simulink model "clock_recovery_4"  (Simulink 7.4)
settings: Solver=ode45  StartTime=0.0  StopTime=1e-5  MaxStep=.1/bit_rate  RelTol=1e-3
PreLoadFcn:
  | bit_rate=2e9;   % bits per second
  | load diff_backplane_model;
undefined symbols (not defined in the file or in its folder): RationalFuncModel
libraries: simulink x8, dspsigattribs x8, dspsigops x6, commblksprivate x4, dspstat3 x2, commrandsrc2 x1, dspbuff3 x1, dspsnks4 x1
settings Model: Creator=dbenson  LastModifiedBy=Dick
settings SolverCC: ZeroCrossControl=EnableAll
settings OptimizationCC: InitFltsAndDblsToZero=on

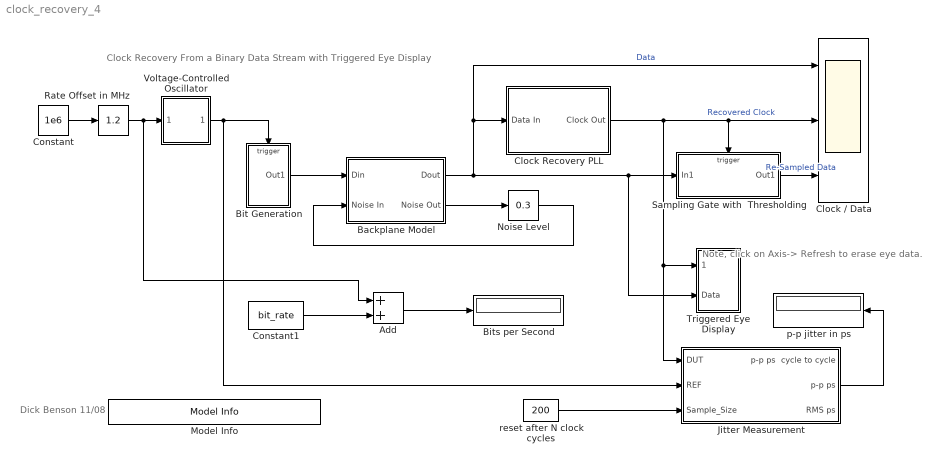
== system clock_recovery_4 ==
  note: Clock Recovery From a Binary Data Stream
      | with
      | Triggered Eye Display
  note: Note, click on Axis-> Refresh
      | to erase eye data.
  note: Dick Benson
      | 11/08
  Add : Sum  OutDataType=sfix(16)  OutScaling=2^-10
  Backplane Model : Subsystem
  Bit Generation : Subsystem
  Bits per Second : Display
  "Clock / Data " : Scope  NumInputPorts=3
      settings: TimeRange=1e-009  YMin=-1~-0.2~-0.2  YMax=1~1.2~1.2
  Clock Recovery PLL : Subsystem
  Constant : Constant  Value=1e6  OutDataType=sfix(16)  OutScaling=2^0
  Constant1 : Constant  Value=bit_rate  OutDataType=sfix(16)  OutScaling=2^0
  "Jitter Measurement " : Subsystem
  Model Info : simulink/Model-Wide Utilities/Model Info  SystemSampleTime=-1  InitialBlockCM=None  BlockCM=None  Frame=on  DisplayStringWithTags=Copywrite 2008-2010 The MathWorks, Inc.  HorizontalTextAlignment=Center  LeftAlignmentValue=0.5  SourceBlockDiagram=clock_recovery_4  TagMaxNumber=20
  Noise Level : simulink/Math Operations/Slider Gain  SystemSampleTime=-1  low=0  gain=0.3  high=1
  Rate Offset in MHz : simulink/Math Operations/Slider Gain  SystemSampleTime=-1  low=-5  gain=1.2  high=5
  Sampling Gate with  Thresholding : Subsystem
  Triggered Eye Display : Subsystem
  Voltage-Controlled Oscillator : Subsystem  mask(Voltage-Controlled Oscillator){Ac=1, Fc=bit_rate, Kc=1, Ph=0}
      mask prompts: Ac "Output amplitude:"; Fc "Oscillation frequency (Hz):"; Kc "Input sensitivity:"; Ph "Initial phase (rad):"
      mask help: Generate a continuous-time output signal whose frequency changes in response to the amplitude variations of the input signal. The input signal must be a sample-based scalar.
      mask init:
      | if ((length(Ac)~=1) | (length(Fc)~=1) | (length(Ph)~=1) | (length(Kc)~=1) )error('Mask parameters must be scalar values.');end;
      | pi2=2*pi;
      mask Help: helpview(commbhelp)
      mask Display: disp('VCO')
  p-p jitter in ps : Display
  reset after N clock cycles : Constant  Value=200  VectorParams1D=off  OutDataType=sfix(16)  OutScaling=2^0
  wires:
  Clock Recovery PLL/1(Clock Out) -> Sampling Gate with  Thresholding/Trigger, "Clock / Data "/2, Triggered Eye Display/1(Trigger), "Jitter Measurement "/1(DUT)  "Recovered Clock"
  Bit Generation/1(Out1) -> Backplane Model/1(Din)
  Backplane Model/1(Dout) -> Clock Recovery PLL/1(Data In), "Clock / Data "/1, Sampling Gate with  Thresholding/1(In1), Triggered Eye Display/2(Data)  "Data"
  Sampling Gate with  Thresholding/1(Out1) -> "Clock / Data "/3  "Re-Sampled Data"
  Add/1 -> Bits per Second/1
  "Jitter Measurement "/2(p-p ps) -> p-p jitter in ps/1
  reset after N clock cycles/1 -> "Jitter Measurement "/3(Sample_Size)
  Backplane Model/2(Noise Out) -> Noise Level/1
  Noise Level/1 -> Backplane Model/2(Noise In)
  Voltage-Controlled Oscillator/1(out_1) -> Bit Generation/Trigger, "Jitter Measurement "/2(REF)
  Rate Offset in MHz/1 -> Voltage-Controlled Oscillator/1(in_1), Add/1
  Constant/1 -> Rate Offset in MHz/1
  Constant1/1 -> Add/2

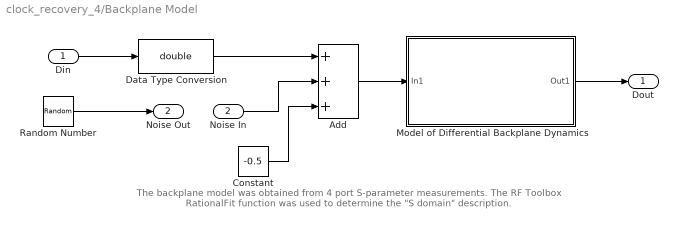
== system clock_recovery_4/Backplane Model ==
  note: The backplane model was obtained from 4 port S-parameter measurements.
      | The RF Toolbox RationalFit function was used to determine the "S domain"
      | description.
  Din : Inport
  Noise In : Inport  Port=2
  Add : Sum  Inputs=+++  OutDataType=sfix(16)  OutScaling=2^-10
  Constant : Constant  Value=-0.5  OutDataType=sfix(16)  OutScaling=2^0
  Data Type Conversion : DataTypeConversion  OutDataTypeMode=double  OutDataType=sfix(16)  OutScaling=2^0  OutDataTypeStr=double
  Model of Differential Backplane Dynamics : Subsystem  mask{RationalFuncModel=RationalFuncModel}
      mask prompts: RationalFuncModel "Rational Model"
      mask init:
      | nPoles = length(RationalFuncModel.A);
      | OriginalA = RationalFuncModel.A; OriginalC = RationalFuncModel.C;
      | A = zeros(length(OriginalA), 1); C = zeros(length(OriginalC), 1);
      | kk = 1;
      | for k = 1:nPoles
      |     if isnan(OriginalA(k))
      |         continue
      |     elseif ~isreal(OriginalA(k))
      |         % Complex poles and residues
      |         pos = find(OriginalA == conj(OriginalA(k)), 1);
      |         OriginalA(pos) = NaN; OriginalC(pos) = NaN;
      |     end
      |     A(kk) = OriginalA(k); C(kk) = OriginalC(k); kk = kk + 1;
      | end
      | A = A(1:kk-1); C = C(1:kk-1);
      | % Get the Numerators and Denominators of the Laplace Transform S-Domain Filters
      | % Convert the vectors of real and complex poles and residues of the rational function model 
      | % into real numerators and denominators of Laplace Transform S-domain filters. 
      | 
      | nA = length(A); 
      | rat_den = cell(nA, 1); 
      | rat_num = cell(nA, 1);
      | 
      | 
      | for k = 1:nA
      |     if isreal(A(k))     % Real poles
      |         rat_num{k} = C(k); rat_den{k} = [1, -A(k)];
      |     else                % Complex poles
      |         real_a = real(A(k)); imag_a = imag(A(k));
      |         real_c = real(C(k)); imag_c = imag(C(k));
      |         rat_num{k} = [2*real_c, -2*(real_a*real_c+imag_a*imag_c)];
      |         rat_den{k} = [1, -2*real_a, real_a^2+imag_a^2];
      |     end
      | end
      | xfer_blocks = length(rat_den);
      | rtsys        = gcb;   % Block become "current" when its initialize function is called.
      | Xfer_stages  = find_system(rtsys,'RegExp','on','lookUnderMasks', 'all', 'FollowLinks','on','BlockType','TransferFcn'); % note there are no spaces in the TransferFcn !!!
      | L_stage = length(Xfer_stages);
      |    %In_port      = find_system(rtsys,'lookUnderMasks', 'all','BlockType','Inport');
      |    %Out_port     = find_system(rtsys,'lookUnderMasks', 'all','BlockType','Outport');
      |    Gain_stage   = find_system(rtsys,'lookUnderMasks', 'all', 'BlockType','Gain');
      |    Sum_stages   = find_system(rtsys,'lookUnderMasks', 'all', 'BlockType','Sum');
      |    Delay_stage  = find_system(rtsys,'lookUnderMasks', 'all', 'BlockType','TransportDelay');
      | 
      | if L_stage ~=nA
      |   %  Delete existing elements (Brute Force!) 
      |    disp('Programatically Building Rational Transfer Function Block ') 
      |   % need to rebuild the model
      |    if L_stage >1
      |        for k=2:L_stage
      |            % need to go in order that is in Xfer_stages
      |            s = Xfer_stages{k};
      |            p = findstr('_',s);
      |            p_last = p(end);
      |            stage=(s((p_last+1):end));
      |            delete_line(rtsys, 'In1/1' , ['stage_',stage,'/1']);
      |            delete_line(rtsys,['stage_',stage,'/1'],['Combiner/',stage]);
      |            % disp(['Deleting ',['stage_',stage]])
      |            delete_block(Xfer_stages{k}); 
      |            drawnow;
      |        end;
      |    end;
      | 
      |    
      |    % set direct feedthrough gain
      |    set_param(Gain_stage{1},'Gain',sprintf('%30d',RationalFuncModel.D)); % the gain value
      |    % set delay element value
      |    % get_param(Delay_stage{1},'ObjectParameters')
      |    set_param(Delay_stage{1},'Delay',sprintf('%30d',RationalFuncModel.Delay)); % delay value
      |    set_param(Delay_stage{1},'BufferSize','2*6144'); % this needs more work ##############
      |    drawnow;
      |    
      |    
      |    % Rebuild structure
      |    % setup combiner (summer) to correct number of inputs
      |    % Set up the Combiner
      |    % get_param(Sum_stages{2},'ObjectParameters')
      |    % get_param(Sum_stages{2},'Inputs')
      |    s='+';
      |    for k=2:xfer_blocks
      |        s=[s,'+'];
      |    end;
      |    set_param(Sum_stages{2},'Inputs',s);  % sets number of inputs to Combiner block
      | 
      |    % add Xfer Fcn blocks
      |    % get_param(Xfer_stages{1},'ObjectParameters')
      |    xfer_pos=get_param(Xfer_stages{1},'Position');
      |    % name_1 = get_param(Xfer_stages{1},'Name');
      |    nstring = ['[',sprintf('%35.5f',rat_num{1}),']'];
      |    dstring = ['[',sprintf('%35.5f',rat_den{1}),']'];
      |    set_param(Xfer_stages{1},'Numerator',nstring,'Denominator',dstring);
      |    src = Xfer_stages{1};  % use as reference block
      |    for k=2:xfer_blocks
      |        dst=[src(1:(end-1)),int2str(k)];
      |        nstring = ['[',sprintf('%35.5f',rat_num{k}),']'];
      |        dstring = ['[',sprintf('%35.5f',rat_den{k}),']'];
      |        add_block(src,dst,'Position',[xfer_pos(1) ,xfer_pos(2)+(k-1)*50, xfer_pos(3) ,xfer_pos(4)+(k-1)*50],'Numerator',nstring,'Denominator',dstring);
      |        add_line(rtsys,'In1/1',['stage_',int2str(k),'/1'],'autorouting','on'); % hook up inputs
      |        add_line(rtsys,['stage_',int2str(k),'/1'],['Combiner/',int2str(k)],'autorouting','on'); % and outputs 
      |     end;
      | 
      | else
      |     % Order has not changed, but coefficients may have.
      |     disp('No programatic build is required, but coefficients are being updated.')
      |     % set direct feedthrough gain
      |     set_param(Gain_stage{1},'Gain',sprintf('%30d',RationalFuncModel.D)); % the gain value
      |     % set delay element value
      |     set_param(Delay_stage{1},'Delay',sprintf('%30d',RationalFuncModel.Delay)); % delay value
      |     set_param(Delay_stage{1},'BufferSize','2*6144'); % this needs more work ##############
      |     
      |     src = Xfer_stages{1};  % use as reference block
      |     for k=1:xfer_blocks
      |        dst=[src(1:(end-1)),int2str(k)];
      |        nstring = ['[',sprintf('%35.5f',rat_num{k}),']'];
      |        dstring = ['[',sprintf('%35.5f',rat_den{k}),']'];
      |        set_param(dst,'Numerator',nstring,'Denominator',dstring); drawnow;
      |     end;
      |         
      | end;
      mask Display: disp('S domain \n Rational Transfer Function Model \n Do Not Edit This Subsystem!')
  Random Number : RandomNumber  SampleTime=0
  Dout : Outport
  Noise Out : Outport  Port=2
  wires:
  Din/1 -> Data Type Conversion/1
  Add/1 -> Model of Differential Backplane Dynamics/1(In1)
  Data Type Conversion/1 -> Add/1
  Model of Differential Backplane Dynamics/1(Out1) -> Dout/1
  Random Number/1 -> Noise Out/1
  Noise In/1 -> Add/2
  Constant/1 -> Add/3

== system clock_recovery_4/Bit Generation ==
  Trigger : TriggerPort
  Bernoulli Binary Generator : commrandsrc2/Bernoulli Binary Generator  DialogController=commDDGCreate  DialogControllerArgs=DataTag0  SystemSampleTime=-1  P=0.5  seed=21  Ts=-1  frameBased=off  sampPerFrame=1  orient=off  outDataType=boolean
  Out1 : Outport
  wires:
  Bernoulli Binary Generator/1 -> Out1/1

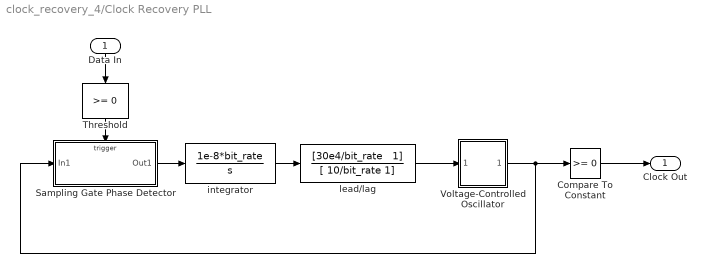
== system clock_recovery_4/Clock Recovery PLL ==
  Data In : Inport
  Compare To Constant : simulink/Logic and Bit Operations/Compare To Constant  SystemSampleTime=-1  relop=>=  const=0  LogicOutDataTypeMode=boolean  ZeroCross=off
  Sampling Gate Phase Detector : Subsystem
  Threshold : simulink/Logic and Bit Operations/Compare To Constant  SystemSampleTime=-1  relop=>=  const=0  LogicOutDataTypeMode=boolean  ZeroCross=off
  Voltage-Controlled Oscillator : Subsystem  mask(Voltage-Controlled Oscillator){Ac=1, Fc=bit_rate, Kc=bit_rate, Ph=0}
      mask prompts: Ac "Output amplitude:"; Fc "Oscillation frequency (Hz):"; Kc "Input sensitivity:"; Ph "Initial phase (rad):"
      mask help: Generate a continuous-time output signal whose frequency changes in response to the amplitude variations of the input signal. The input signal must be a sample-based scalar.
      mask init:
      | if ((length(Ac)~=1) | (length(Fc)~=1) | (length(Ph)~=1) | (length(Kc)~=1) )error('Mask parameters must be scalar values.');end;
      | pi2=2*pi;
      mask Help: helpview(commbhelp)
      mask Display: disp('VCO')
  integrator : TransferFcn  Numerator=1e-8*bit_rate  Denominator=[1 0]
  lead/lag : TransferFcn  Numerator="[30e4/bit_rate   1]"  Denominator=[ 10/bit_rate 1]
  Clock Out : Outport
  wires:
  lead/lag/1 -> Voltage-Controlled Oscillator/1(in_1)
  Voltage-Controlled Oscillator/1(out_1) -> Sampling Gate Phase Detector/1(In1), Compare To Constant/1
  integrator/1 -> lead/lag/1
  Sampling Gate Phase Detector/1(Out1) -> integrator/1
  Threshold/1 -> Sampling Gate Phase Detector/Trigger
  Data In/1 -> Threshold/1
  Compare To Constant/1 -> Clock Out/1

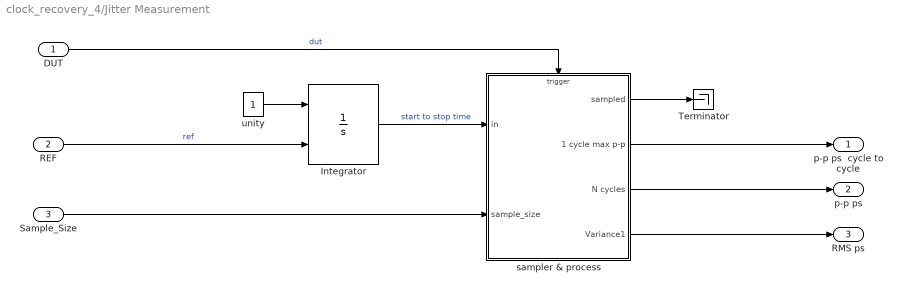
== system clock_recovery_4/Jitter Measurement  ==
  DUT : Inport  OutDataType=sfix(16)  OutScaling=2^0
  REF : Inport  Port=2  OutDataType=sfix(16)  OutScaling=2^0
  Sample_Size : Inport  Port=3  OutDataType=sfix(16)  OutScaling=2^0
  Integrator : Integrator  ExternalReset=rising
  Terminator : Terminator
  sampler & process : Subsystem  TreatAsAtomicUnit=on
  unity : Constant  OutDataTypeMode=double  OutDataType=sfix(16)  OutScaling=2^0  OutDataTypeStr=double
  p-p ps  cycle to cycle : Outport  OutDataType=sfix(16)  OutScaling=2^0
  p-p ps : Outport  Port=2  OutDataType=sfix(16)  OutScaling=2^0
  RMS ps : Outport  Port=3  OutDataType=sfix(16)  OutScaling=2^0
  wires:
  DUT/1 -> sampler & process/Trigger  "dut"
  REF/1 -> Integrator/2  "ref"
  Integrator/1 -> sampler & process/1(in)  "start to stop time"
  Sample_Size/1 -> sampler & process/2(sample_size)
  sampler & process/3(N cycles) -> p-p ps/1
  sampler & process/4(Variance1) -> RMS ps/1
  unity/1 -> Integrator/1
  sampler & process/2(1 cycle max p-p) -> p-p ps  cycle to cycle/1
  sampler & process/1(sampled) -> Terminator/1

== system clock_recovery_4/Sampling Gate with  Thresholding ==
  In1 : Inport  OutDataType=sfix(16)  OutScaling=2^0
  Trigger : TriggerPort
  Compare To Constant : simulink/Logic and Bit Operations/Compare To Constant  SystemSampleTime=-1  relop=>=  const=0  LogicOutDataTypeMode=boolean  ZeroCross=off
  Out1 : Outport  OutDataType=sfix(16)  OutScaling=2^0
  wires:
  In1/1 -> Compare To Constant/1
  Compare To Constant/1 -> Out1/1

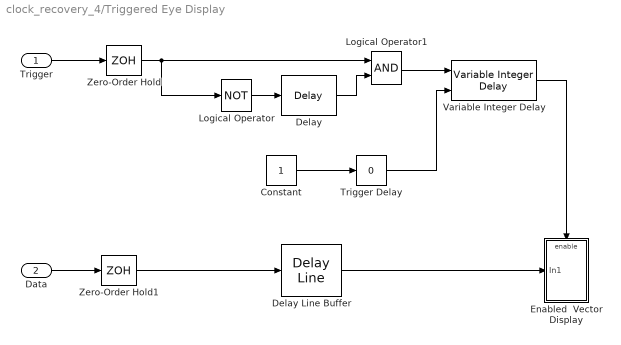
== system clock_recovery_4/Triggered Eye Display ==
  Trigger : Inport
  Data : Inport  Port=2
  Constant : Constant  OutDataType=sfix(16)  OutScaling=2^0
  Delay : dspsigops/Delay  dly_unit=Samples  delay=1  ic_detail=off  dif_ic_for_ch=off  dif_ic_for_dly=off  ic=0  reset_popup=None
  Delay Line Buffer : dspbuff3/Delay Line  siz=200  ic=0  directfeed=off  enable_output=off  hold_output=off
  Enabled  Vector Display : Subsystem
  Logical Operator : Logic  Operator=NOT  AllPortsSameDT=off  OutDataTypeMode=boolean  OutDataTypeStr=boolean
  Logical Operator1 : Logic  AllPortsSameDT=off  OutDataTypeMode=boolean  OutDataTypeStr=boolean
  Trigger Delay : simulink/Math Operations/Slider Gain  SystemSampleTime=-1  low=0  gain=0  high=100
  Variable Integer Delay : dspsigops/Variable Integer Delay  dmax=100  ic=0  noDFT=off
  Zero-Order Hold : ZeroOrderHold  SampleTime=.01/bit_rate
  Zero-Order Hold1 : ZeroOrderHold  SampleTime=.01/bit_rate
  wires:
  Zero-Order Hold/1 -> Logical Operator1/1, Logical Operator/1
  Logical Operator/1 -> Delay/1
  Delay/1 -> Logical Operator1/2
  Trigger/1 -> Zero-Order Hold/1
  Data/1 -> Zero-Order Hold1/1
  Zero-Order Hold1/1 -> Delay Line Buffer/1
  Delay Line Buffer/1 -> Enabled  Vector Display/1(In1)
  Logical Operator1/1 -> Variable Integer Delay/1
  Variable Integer Delay/1 -> Enabled  Vector Display/Enable
  Trigger Delay/1 -> Variable Integer Delay/2
  Constant/1 -> Trigger Delay/1

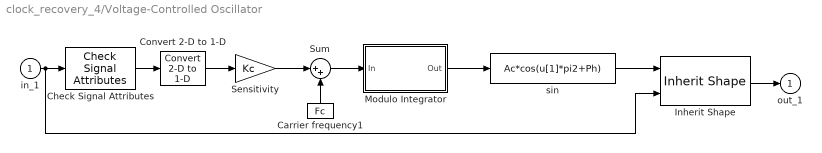
== system clock_recovery_4/Voltage-Controlled Oscillator ==
  in_1 : Inport  OutDataType=sfix(16)  OutScaling=2^0
  Carrier frequency1 : Constant  Value=Fc  OutDataType=sfix(16)  OutScaling=2^0
  Check Signal Attributes : dspsigattribs/Check Signal Attributes  SystemSampleTime=-1  SigAttribCheckMethod=Does not match attributes exactly  Complexity=Ignore  Frame=Sample-based  DimsCheckMethod=Is...  Dimensions=Scalar (1-D or 2-D)  DatatypeCheckMethod=Ignore  DatatypeGeneral=Boolean  DtypeFloatSpecific=Any floating-point  DtypeFixedSpecific=Any fixed-point  DtypeIntSpecific=Any integer  SampleMode=Ignore
  Convert 2-D to 1-D : dspsigattribs/Convert 2-D to 1-D  SystemSampleTime=-1
  Inherit Shape : commblksprivate/Inherit Shape
  Modulo Integrator : Subsystem  mask(Modulo Integrator){modu=1, init=0}
      mask prompts: modu "Absolute value bound:"; init "Initial condition:"
      mask help:
      | Integrate the input signal in continuous time and then uses the Absolute value bound parameter, K, to produce output strictly between -K and K. The block uses the rem function in MATLAB.
      |
      | The input must be sample-based.
      mask init:
      | [modu, init]=commblkmodint(gcb);
      mask Help: helpview(commbhelp)
      mask Display: disp('Modulo\nIntegrator')
  Sensitivity : Gain  Gain=Kc  ParameterDataType=sfix(16)  ParameterScaling=2^0  OutDataType=sfix(16)  OutScaling=2^0  SaturateOnIntegerOverflow=on  OutDataTypeStr=Inherit: Same as input  ParamDataTypeStr=Inherit: Same as input
  Sum : Sum  Inputs=|++  OutDataType=sfix(16)  OutScaling=2^0  SaturateOnIntegerOverflow=on  InputSameDT=on  OutDataTypeStr=Inherit: Same as first input
  sin : Fcn  Expr=Ac*cos(u[1]*pi2+Ph)
  out_1 : Outport  OutDataType=sfix(16)  OutScaling=2^0  InitialOutput=0
  wires:
  Check Signal Attributes/1 -> Convert 2-D to 1-D/1
  Inherit Shape/1 -> out_1/1
  sin/1 -> Inherit Shape/1
  Convert 2-D to 1-D/1 -> Sensitivity/1
  in_1/1 -> Check Signal Attributes/1, Inherit Shape/2
  Sensitivity/1 -> Sum/1
  Carrier frequency1/1 -> Sum/2
  Modulo Integrator/1(Out) -> sin/1
  Sum/1 -> Modulo Integrator/1(In)

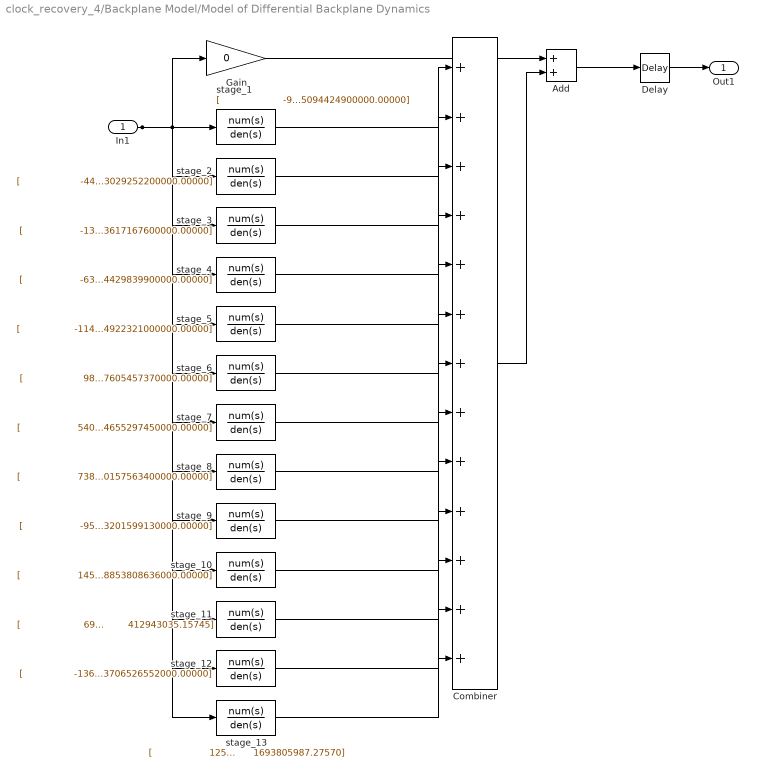
== system clock_recovery_4/Backplane Model/Model of Differential Backplane Dynamics ==
  In1 : Inport  OutDataType=sfix(16)  OutScaling=2^0
  Add : Sum  OutDataType=sfix(16)  OutScaling=2^-10
  Combiner : Sum  Inputs=+++++++++++++  OutDataType=sfix(16)  OutScaling=2^-10
  Delay : TransportDelay  DelayTime=5.950332e-009  BufferSize=2*6144
  Gain : Gain  Gain=0  ParameterDataType=sfix(16)  ParameterScaling=2^0  OutDataType=sfix(16)  OutScaling=2^0
  stage_1 : TransferFcn  Numerator="[                     -9788555.30433           327601364005149500.00000]"  Denominator="[                            1.00000                   1329591272.34003       5044242645094424900000.00000]"
  stage_10 : TransferFcn  Numerator="[                   1459155273.40124         16659733674469984000.00000]"  Denominator="[                            1.00000                   4539756715.10415         55819688853808636000.00000]"
  stage_11 : TransferFcn  Numerator="[                     69890645.34105]"  Denominator="[                            1.00000                    412943035.15745]"
  stage_12 : TransferFcn  Numerator="[                 -13652042138.80265        -20558972237464187000.00000]"  Denominator="[                            1.00000                   6618433668.53674         16544543706526552000.00000]"
  stage_13 : TransferFcn  Numerator="[                   1252271665.41653]"  Denominator="[                            1.00000                   1693805987.27570]"
  stage_2 : TransferFcn  Numerator="[                    -44020735.77568          2540524038618086400.00000]"  Denominator="[                            1.00000                   3458566159.00361       3748760873029252200000.00000]"
  stage_3 : TransferFcn  Numerator="[                   -134087089.17792          1299068138817301200.00000]"  Denominator="[                            1.00000                   4003736859.07552       2889729443617167600000.00000]"
  stage_4 : TransferFcn  Numerator="[                   -637966669.86598         -4277202848730946600.00000]"  Denominator="[                            1.00000                   7795187757.93497       1980584994429839900000.00000]"
  stage_5 : TransferFcn  Numerator="[                  -1141903615.08100        -42517650479109677000.00000]"  Denominator="[                            1.00000                   6993651024.28011       1349862304922321000000.00000]"
  stage_6 : TransferFcn  Numerator="[                    985358456.83414        -87067793597322330000.00000]"  Denominator="[                            1.00000                   7852217292.40317        928900427605457370000.00000]"
  stage_7 : TransferFcn  Numerator="[                   5400452167.19306        -32568397331195798000.00000]"  Denominator="[                            1.00000                   8411433569.92250        523163784655297450000.00000]"
  stage_8 : TransferFcn  Numerator="[                   7386311262.49890        115624507669340000000.00000]"  Denominator="[                            1.00000                   7724253224.87238        259580420157563400000.00000]"
  stage_9 : TransferFcn  Numerator="[                   -952042760.73716         71238284461090677000.00000]"  Denominator="[                            1.00000                   6002589292.72624        101064183201599130000.00000]"
  Out1 : Outport  OutDataType=sfix(16)  OutScaling=2^0
  wires:
  In1/1 -> Gain/1, stage_1/1, stage_2/1, stage_3/1, stage_4/1, stage_5/1, stage_6/1, stage_7/1, stage_8/1, stage_9/1, stage_10/1, stage_11/1, stage_12/1, stage_13/1
  Gain/1 -> Add/1
  Add/1 -> Delay/1
  Combiner/1 -> Add/2
  Delay/1 -> Out1/1
  stage_1/1 -> Combiner/1
  stage_2/1 -> Combiner/2
  stage_3/1 -> Combiner/3
  stage_4/1 -> Combiner/4
  stage_5/1 -> Combiner/5
  stage_6/1 -> Combiner/6
  stage_7/1 -> Combiner/7
  stage_8/1 -> Combiner/8
  stage_9/1 -> Combiner/9
  stage_10/1 -> Combiner/10
  stage_11/1 -> Combiner/11
  stage_12/1 -> Combiner/12
  stage_13/1 -> Combiner/13

== system clock_recovery_4/Clock Recovery PLL/Sampling Gate Phase Detector ==
  In1 : Inport  OutDataType=sfix(16)  OutScaling=2^0
  Trigger : TriggerPort
  Out1 : Outport  OutDataType=sfix(16)  OutScaling=2^0
  wires:
  In1/1 -> Out1/1

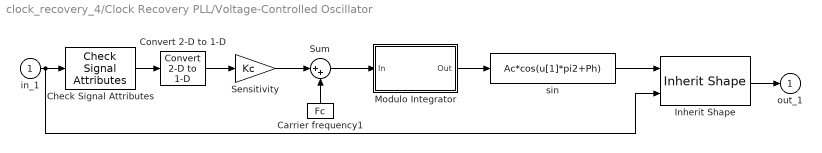
== system clock_recovery_4/Clock Recovery PLL/Voltage-Controlled Oscillator ==
  in_1 : Inport  OutDataType=sfix(16)  OutScaling=2^0
  Carrier frequency1 : Constant  Value=Fc  OutDataType=sfix(16)  OutScaling=2^0
  Check Signal Attributes : dspsigattribs/Check Signal Attributes  SystemSampleTime=-1  SigAttribCheckMethod=Does not match attributes exactly  Complexity=Ignore  Frame=Sample-based  DimsCheckMethod=Is...  Dimensions=Scalar (1-D or 2-D)  DatatypeCheckMethod=Ignore  DatatypeGeneral=Boolean  DtypeFloatSpecific=Any floating-point  DtypeFixedSpecific=Any fixed-point  DtypeIntSpecific=Any integer  SampleMode=Ignore
  Convert 2-D to 1-D : dspsigattribs/Convert 2-D to 1-D  SystemSampleTime=-1
  Inherit Shape : commblksprivate/Inherit Shape
  Modulo Integrator : Subsystem  mask(Modulo Integrator){modu=1, init=0}
      mask prompts: modu "Absolute value bound:"; init "Initial condition:"
      mask help:
      | Integrate the input signal in continuous time and then uses the Absolute value bound parameter, K, to produce output strictly between -K and K. The block uses the rem function in MATLAB.
      |
      | The input must be sample-based.
      mask init:
      | [modu, init]=commblkmodint(gcb);
      mask Help: helpview(commbhelp)
      mask Display: disp('Modulo\nIntegrator')
  Sensitivity : Gain  Gain=Kc  ParameterDataType=sfix(16)  ParameterScaling=2^0  OutDataType=sfix(16)  OutScaling=2^0  SaturateOnIntegerOverflow=on  OutDataTypeStr=Inherit: Same as input  ParamDataTypeStr=Inherit: Same as input
  Sum : Sum  Inputs=|++  OutDataType=sfix(16)  OutScaling=2^0  SaturateOnIntegerOverflow=on  InputSameDT=on  OutDataTypeStr=Inherit: Same as first input
  sin : Fcn  Expr=Ac*cos(u[1]*pi2+Ph)
  out_1 : Outport  OutDataType=sfix(16)  OutScaling=2^0  InitialOutput=0
  wires:
  Check Signal Attributes/1 -> Convert 2-D to 1-D/1
  Inherit Shape/1 -> out_1/1
  sin/1 -> Inherit Shape/1
  Convert 2-D to 1-D/1 -> Sensitivity/1
  in_1/1 -> Check Signal Attributes/1, Inherit Shape/2
  Sensitivity/1 -> Sum/1
  Carrier frequency1/1 -> Sum/2
  Modulo Integrator/1(Out) -> sin/1
  Sum/1 -> Modulo Integrator/1(In)

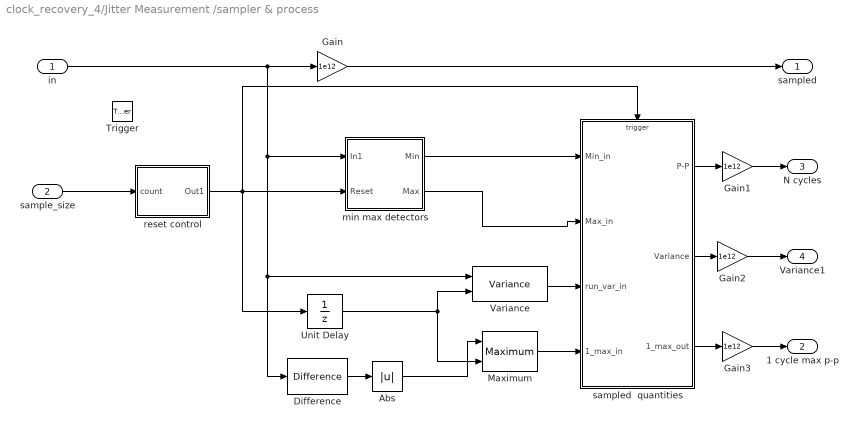
== system clock_recovery_4/Jitter Measurement /sampler & process ==
  in : Inport  OutDataType=sfix(16)  OutScaling=2^0
  sample_size : Inport  Port=2  OutDataType=sfix(16)  OutScaling=2^0
  Trigger : TriggerPort
  Abs : Abs
  Difference : simulink/Discrete/Difference  SystemSampleTime=-1  ICPrevInput=0.0  OutMin=[]  OutMax=[]  OutDataType=sfix(16)  OutScaling=2^-10  DoSatur=off
  Gain{,1..3} (4 alike) : Gain  Gain=1e12  ParameterDataType=sfix(16)  ParameterScaling=2^0  OutDataType=sfix(16)  OutScaling=2^0
  Maximum : dspstat3/Maximum  DialogController=dspDDGCreate  DialogControllerArgs=DataTag1  fcn=Running  reset=Rising edge  indexBase=One  operateOver=Each column  Dimension=1  colComp=on  operation=maximum  roiEnable=off  roiType=Rectangles  roiPortion=Entire ROI  roiOutput=Individual statistics for each ROI  roiFlag=off  accumDataTypeStr=Inherit: Same as product output  accumLastDataTypeStr=Inherit: Same as product output  roundingMode=Floor  overflowMode=off
  Unit Delay : UnitDelay  SampleTime=-1
  Variance : dspstat3/Variance  DialogController=dspDDGCreate  DialogControllerArgs=DataTag2  run=on  reset_popup=Rising edge  directionMode=Each column  dimension=1  treatSBRowAsCol=on  roiEnable=off  roiType=Rectangles  roiPortion=Entire ROI  roiOutput=Individual statistics for each ROI  roiFlag=off  roundingMode=Floor  overflowMode=off
  min max detectors : Subsystem
  reset control : Subsystem
  sampled  quantities : Subsystem  TreatAsAtomicUnit=on
  sampled : Outport  OutDataType=sfix(16)  OutScaling=2^0
  1 cycle max p-p : Outport  Port=2  OutDataType=sfix(16)  OutScaling=2^0
  N cycles : Outport  Port=3  OutDataType=sfix(16)  OutScaling=2^0
  Variance1 : Outport  Port=4  OutDataType=sfix(16)  OutScaling=2^0
  wires:
  in/1 -> Gain/1, Variance/1, Difference/1, min max detectors/1(In1)
  Difference/1 -> Abs/1
  Abs/1 -> Maximum/1
  sample_size/1 -> reset control/1(count)
  reset control/1(Out1) -> Unit Delay/1, sampled  quantities/Trigger, min max detectors/2(Reset)
  sampled  quantities/1(P-P) -> Gain1/1
  Variance/1 -> sampled  quantities/3(run_var_in)
  sampled  quantities/2(Variance) -> Gain2/1
  Unit Delay/1 -> Variance/2, Maximum/2
  Maximum/1 -> sampled  quantities/4(1_max_in)
  sampled  quantities/3(1_max_out) -> Gain3/1
  Gain/1 -> sampled/1
  Gain1/1 -> N cycles/1
  Gain2/1 -> Variance1/1
  Gain3/1 -> 1 cycle max p-p/1
  min max detectors/2(Max) -> sampled  quantities/2(Max_in)
  min max detectors/1(Min) -> sampled  quantities/1(Min_in)

== system clock_recovery_4/Triggered Eye Display/Enabled  Vector Display ==
  In1 : Inport
  Enable : EnablePort
  Vector Scope1 : dspsnks4/Vector Scope  DialogController=dspdialog.VectorScope  DialogControllerArgs=DataTag3  ScopeProperties=on  Domain=User-defined  HorizSpan=1  DisplayProperties=off  AxisGrid=on  Memory=on  FrameNumber=on  AxisLegend=off  AxisZoom=off  OpenScopeAtSimStart=on  OpenScopeImmediately=off  FigPos=[3 39 417 270]  AxisProperties=off  XUnits=Hertz  XRange=[0...Fs/2]  InheritXIncr=off  XIncr=.01/bit_rate  XLabel=Time  XLimit=Auto  XMin=0  XMax=1  XStart=0  YUnits=dB  YLabel=Amplitude  LineProperties=off  LineColors=[0 0 1]|[1 0 0]  XAxisParamsVer=6.8
      settings: YMin=-.7  YMax=.7
  wires:
  In1/1 -> Vector Scope1/1

== system clock_recovery_4/Voltage-Controlled Oscillator/Modulo Integrator ==
  In : Inport  OutDataType=sfix(16)  OutScaling=2^0
  "Exclude Frame-based Input " : dspsigattribs/Check Signal Attributes  SystemSampleTime=-1  SigAttribCheckMethod=Matches attributes exactly  Complexity=Ignore  Frame=Frame-based  DimsCheckMethod=Ignore  Dimensions=Scalar (1-D or 2-D)  DatatypeCheckMethod=Ignore  DatatypeGeneral=Boolean  DtypeFloatSpecific=Any floating-point  DtypeFixedSpecific=Any fixed-point  DtypeIntSpecific=Any integer  SampleMode=Ignore
  Exclude Full Matrix : dspsigattribs/Check Signal Attributes  SystemSampleTime=-1  SigAttribCheckMethod=Matches attributes exactly  Complexity=Ignore  Frame=Ignore  DimsCheckMethod=Is...  Dimensions=Full matrix (2-D)  DatatypeCheckMethod=Ignore  DatatypeGeneral=Boolean  DtypeFloatSpecific=Any floating-point  DtypeFixedSpecific=Any fixed-point  DtypeIntSpecific=Any integer  SampleMode=Ignore
  Inherit Shape : commblksprivate/Inherit Shape
  Modulo Integrator : Subsystem
  Out : Outport  OutDataType=sfix(16)  OutScaling=2^0
  wires:
  Exclude Full Matrix/1 -> "Exclude Frame-based Input "/1
  "Exclude Frame-based Input "/1 -> Modulo Integrator/1(In1)
  In/1 -> Exclude Full Matrix/1, Inherit Shape/2
  Modulo Integrator/1(Out1) -> Inherit Shape/1
  Inherit Shape/1 -> Out/1

== system clock_recovery_4/Clock Recovery PLL/Voltage-Controlled Oscillator/Modulo Integrator ==
  In : Inport  OutDataType=sfix(16)  OutScaling=2^0
  "Exclude Frame-based Input " : dspsigattribs/Check Signal Attributes  SystemSampleTime=-1  SigAttribCheckMethod=Matches attributes exactly  Complexity=Ignore  Frame=Frame-based  DimsCheckMethod=Ignore  Dimensions=Scalar (1-D or 2-D)  DatatypeCheckMethod=Ignore  DatatypeGeneral=Boolean  DtypeFloatSpecific=Any floating-point  DtypeFixedSpecific=Any fixed-point  DtypeIntSpecific=Any integer  SampleMode=Ignore
  Exclude Full Matrix : dspsigattribs/Check Signal Attributes  SystemSampleTime=-1  SigAttribCheckMethod=Matches attributes exactly  Complexity=Ignore  Frame=Ignore  DimsCheckMethod=Is...  Dimensions=Full matrix (2-D)  DatatypeCheckMethod=Ignore  DatatypeGeneral=Boolean  DtypeFloatSpecific=Any floating-point  DtypeFixedSpecific=Any fixed-point  DtypeIntSpecific=Any integer  SampleMode=Ignore
  Inherit Shape : commblksprivate/Inherit Shape
  Modulo Integrator : Subsystem
  Out : Outport  OutDataType=sfix(16)  OutScaling=2^0
  wires:
  Exclude Full Matrix/1 -> "Exclude Frame-based Input "/1
  "Exclude Frame-based Input "/1 -> Modulo Integrator/1(In1)
  In/1 -> Exclude Full Matrix/1, Inherit Shape/2
  Modulo Integrator/1(Out1) -> Inherit Shape/1
  Inherit Shape/1 -> Out/1

== system clock_recovery_4/Jitter Measurement /sampler & process/min max detectors ==
  In1 : Inport  OutDataType=sfix(16)  OutScaling=2^0
  Reset : Inport  Port=2  OutDataType=sfix(16)  OutScaling=2^0
  Delay1 : dspsigops/Delay  dly_unit=Samples  delay=1  ic_detail=off  dif_ic_for_ch=off  dif_ic_for_dly=off  ic=0  reset_popup=None
  Delay2 : dspsigops/Delay  dly_unit=Samples  delay=1  ic_detail=off  dif_ic_for_ch=off  dif_ic_for_dly=off  ic=0  reset_popup=None
  min_1 : Subsystem
  min_2 : Subsystem
  Min : Outport  OutDataType=sfix(16)  OutScaling=2^0
  Max : Outport  Port=2  OutDataType=sfix(16)  OutScaling=2^0
  wires:
  Reset/1 -> min_1/2(Rst), min_2/2(Rst)
  In1/1 -> min_1/1(In), min_2/1(In)
  min_1/1(Out) -> Delay1/1
  min_2/1(Out) -> Delay2/1
  Delay1/1 -> Min/1
  Delay2/1 -> Max/1

== system clock_recovery_4/Jitter Measurement /sampler & process/reset control ==
  count : Inport  OutDataType=sfix(16)  OutScaling=2^0
  Constant2 : Constant  OutDataType=sfix(16)  OutScaling=2^0
  Fcn4 : Fcn  Expr=u<1
  Math Function : Math  Operator=mod  OutDataType=sfix(16)  OutScaling=2^0  SaturateOnIntegerOverflow=on
  Sum2 : Sum  Inputs=|++  OutDataType=sfix(16)  OutScaling=2^0  SaturateOnIntegerOverflow=on  InputSameDT=on  OutDataTypeStr=Inherit: Same as first input
  Unit Delay1 : UnitDelay  SampleTime=-1
  Out1 : Outport  OutDataType=sfix(16)  OutScaling=2^0
  wires:
  Math Function/1 -> Fcn4/1, Sum2/2
  Unit Delay1/1 -> Math Function/1
  Constant2/1 -> Sum2/1
  Sum2/1 -> Unit Delay1/1
  Fcn4/1 -> Out1/1
  count/1 -> Math Function/2

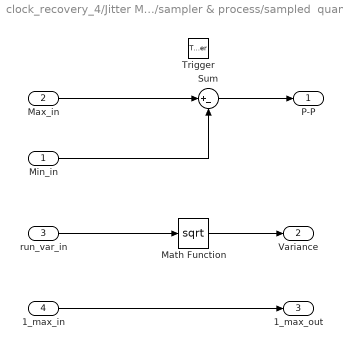
== system clock_recovery_4/Jitter Measurement /sampler & process/sampled  quantities ==
  Min_in : Inport  OutDataType=sfix(16)  OutScaling=2^0
  Max_in : Inport  Port=2  OutDataType=sfix(16)  OutScaling=2^0
  run_var_in : Inport  Port=3  OutDataType=sfix(16)  OutScaling=2^0
  1_max_in : Inport  Port=4  OutDataType=sfix(16)  OutScaling=2^0
  Trigger : TriggerPort
  Math Function : Math  Operator=sqrt  OutDataType=sfix(16)  OutScaling=2^0  SaturateOnIntegerOverflow=on
  Sum : Sum  Inputs=|+-  OutDataType=sfix(16)  OutScaling=2^0  SaturateOnIntegerOverflow=on  InputSameDT=on  OutDataTypeStr=Inherit: Same as first input
  P-P : Outport  OutDataType=sfix(16)  OutScaling=2^0
  Variance : Outport  Port=2  OutDataType=sfix(16)  OutScaling=2^0
  1_max_out : Outport  Port=3  OutDataType=sfix(16)  OutScaling=2^0
  wires:
  Max_in/1 -> Sum/1
  Min_in/1 -> Sum/2
  Sum/1 -> P-P/1
  Math Function/1 -> Variance/1
  run_var_in/1 -> Math Function/1
  1_max_in/1 -> 1_max_out/1

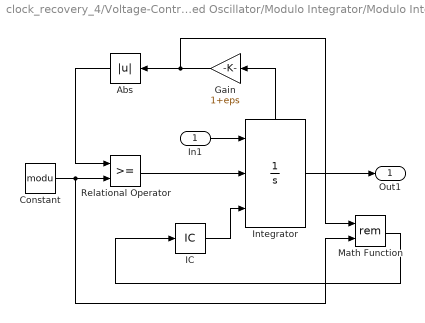
== system clock_recovery_4/Voltage-Controlled Oscillator/Modulo Integrator/Modulo Integrator ==
  In1 : Inport  OutDataType=sfix(16)  OutScaling=2^0
  Abs : Abs  OutDataType=sfix(16)  OutScaling=2^0  SaturateOnIntegerOverflow=on
  Constant : Constant  Value=modu  OutDataType=sfix(16)  OutScaling=2^0
  Gain : Gain  Gain=1+eps  ParameterDataType=sfix(16)  ParameterScaling=2^0  OutDataType=sfix(16)  OutScaling=2^0  SaturateOnIntegerOverflow=on  OutDataTypeStr=Inherit: Same as input  ParamDataTypeStr=Inherit: Same as input
  IC : InitialCondition  Value=init
  Integrator : Integrator  ExternalReset=rising  InitialConditionSource=external  UpperSaturationLimit=1  LowerSaturationLimit=0  ShowStatePort=on
  Math Function : Math  Operator=rem  OutDataType=sfix(16)  OutScaling=2^0  SaturateOnIntegerOverflow=on
  Relational Operator : RelationalOperator  InputSameDT=on
  Out1 : Outport  OutDataType=sfix(16)  OutScaling=2^0
  wires:
  IC/1 -> Integrator/3
  In1/1 -> Integrator/1
  Integrator/1 -> Out1/1
  Math Function/1 -> IC/1
  Abs/1 -> Relational Operator/1
  Relational Operator/1 -> Integrator/2
  Constant/1 -> Math Function/2, Relational Operator/2
  Integrator/State -> Gain/1
  Gain/1 -> Abs/1, Math Function/1

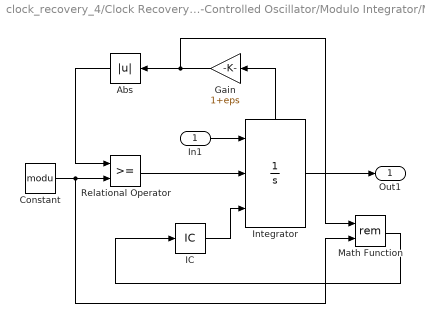
== system clock_recovery_4/Clock Recovery PLL/Voltage-Controlled Oscillator/Modulo Integrator/Modulo Integrator ==
  In1 : Inport  OutDataType=sfix(16)  OutScaling=2^0
  Abs : Abs  OutDataType=sfix(16)  OutScaling=2^0  SaturateOnIntegerOverflow=on
  Constant : Constant  Value=modu  OutDataType=sfix(16)  OutScaling=2^0
  Gain : Gain  Gain=1+eps  ParameterDataType=sfix(16)  ParameterScaling=2^0  OutDataType=sfix(16)  OutScaling=2^0  SaturateOnIntegerOverflow=on  OutDataTypeStr=Inherit: Same as input  ParamDataTypeStr=Inherit: Same as input
  IC : InitialCondition  Value=init
  Integrator : Integrator  ExternalReset=rising  InitialConditionSource=external  UpperSaturationLimit=1  LowerSaturationLimit=0  ShowStatePort=on
  Math Function : Math  Operator=rem  OutDataType=sfix(16)  OutScaling=2^0  SaturateOnIntegerOverflow=on
  Relational Operator : RelationalOperator  InputSameDT=on
  Out1 : Outport  OutDataType=sfix(16)  OutScaling=2^0
  wires:
  IC/1 -> Integrator/3
  In1/1 -> Integrator/1
  Integrator/1 -> Out1/1
  Math Function/1 -> IC/1
  Abs/1 -> Relational Operator/1
  Relational Operator/1 -> Integrator/2
  Constant/1 -> Math Function/2, Relational Operator/2
  Integrator/State -> Gain/1
  Gain/1 -> Abs/1, Math Function/1

== system clock_recovery_4/Jitter Measurement /sampler & process/min max detectors/min_1 ==
  In : Inport  OutDataType=sfix(16)  OutScaling=2^0
  Rst : Inport  Port=2  OutDataType=sfix(16)  OutScaling=2^0
  Delay : dspsigops/Delay  dly_unit=Samples  delay=1  ic_detail=off  dif_ic_for_ch=off  dif_ic_for_dly=off  ic=1e6  reset_popup=Non-zero sample
  Relational Operator : RelationalOperator  Operator=<  LogicOutDataTypeMode=boolean  OutDataTypeStr=boolean
  Switch : Switch  Threshold=.5
  Out : Outport  OutDataType=sfix(16)  OutScaling=2^0
  wires:
  In/1 -> Relational Operator/1, Switch/1
  Rst/1 -> Delay/2
  Delay/1 -> Relational Operator/2, Switch/3
  Relational Operator/1 -> Switch/2
  Switch/1 -> Delay/1, Out/1

== system clock_recovery_4/Jitter Measurement /sampler & process/min max detectors/min_2 ==
  In : Inport  OutDataType=sfix(16)  OutScaling=2^0
  Rst : Inport  Port=2  OutDataType=sfix(16)  OutScaling=2^0
  Delay : dspsigops/Delay  dly_unit=Samples  delay=1  ic_detail=off  dif_ic_for_ch=off  dif_ic_for_dly=off  ic=-1e6  reset_popup=Non-zero sample
  Relational Operator : RelationalOperator  Operator=>  LogicOutDataTypeMode=boolean  OutDataTypeStr=boolean
  Switch : Switch  Threshold=.5
  Out : Outport  OutDataType=sfix(16)  OutScaling=2^0
  wires:
  Switch/1 -> Out/1, Delay/1
  Relational Operator/1 -> Switch/2
  Delay/1 -> Switch/3, Relational Operator/2
  Rst/1 -> Delay/2
  In/1 -> Switch/1, Relational Operator/1
